simulink model "test_simulink"  (R2017a)
settings: Solver=VariableStepAuto  StartTime=0.0  StopTime=10.0  RelTol=1e-3
values from neighbouring files (symbols this model uses):
  ddq = u(15:21)    [accelerations_simulink.m]    (also in comparison_simulink.m = ADAMS_yout(:,37:43); gravity_force_simulink.m; gravity_moment_simulink.m; inertia_force_simulink.m)
settings Model: Creator=ashwi  LastModifiedBy=ashwi

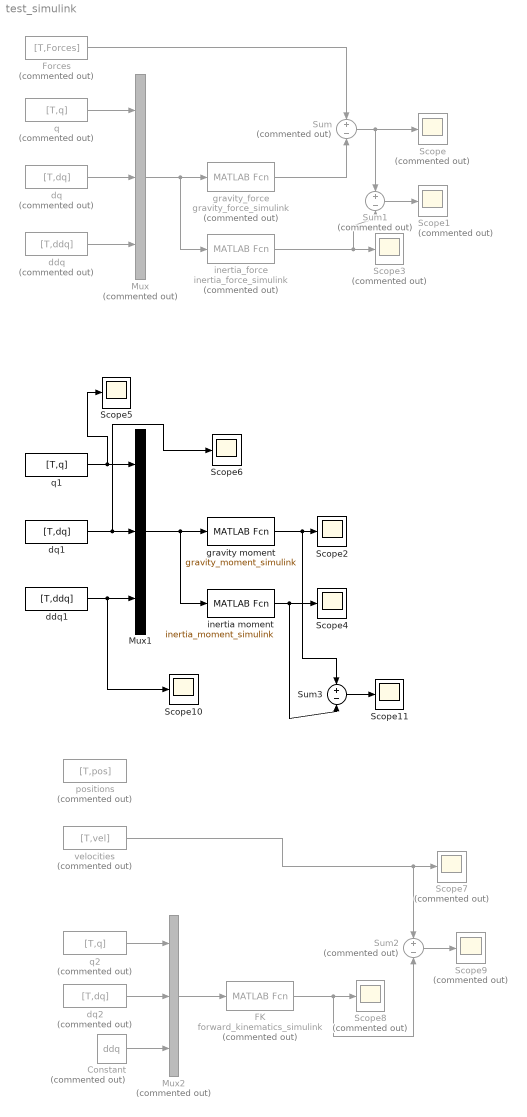
== system test_simulink ==
  Constant : Constant  Commented=on  Value=ddq
  FK : MATLABFcn  Commented=on  MATLABFcn=forward_kinematics_simulink
  Forces : FromWorkspace  Commented=on  VariableName=[T,Forces]  SampleTime=0
  Mux : Mux  Commented=on  Inputs=3
  Mux1 : Mux  Inputs=3
  Mux2 : Mux  Commented=on  Inputs=3
  Scope{,1,3,7..9} (6 alike) : Scope  Commented=on
  Scope{2,4..6,10..11} (6 alike) : Scope
  Sum : Sum  Commented=on  Inputs=+-
  Sum1 : Sum  Commented=on  Inputs=+-
  Sum2 : Sum  Commented=on  Inputs=+-
  Sum3 : Sum  Inputs=+-
  ddq : FromWorkspace  Commented=on  VariableName=[T,ddq]  SampleTime=0
  ddq1 : FromWorkspace  VariableName=[T,ddq]  SampleTime=0
  dq : FromWorkspace  Commented=on  VariableName=[T,dq]  SampleTime=0
  dq1 : FromWorkspace  VariableName=[T,dq]  SampleTime=0
  dq2 : FromWorkspace  Commented=on  VariableName=[T,dq]  SampleTime=0
  gravity moment : MATLABFcn  MATLABFcn=gravity_moment_simulink
  gravity_force : MATLABFcn  Commented=on  MATLABFcn=gravity_force_simulink
  inertia moment : MATLABFcn  MATLABFcn=inertia_moment_simulink
  inertia_force : MATLABFcn  Commented=on  MATLABFcn=inertia_force_simulink
  positions : FromWorkspace  Commented=on  VariableName=[T,pos]  SampleTime=0
  q : FromWorkspace  Commented=on  VariableName=[T,q]  SampleTime=0
  q1 : FromWorkspace  VariableName=[T,q]  SampleTime=0
  q2 : FromWorkspace  Commented=on  VariableName=[T,q]  SampleTime=0
  velocities : FromWorkspace  Commented=on  VariableName=[T,vel]  SampleTime=0
  wires:
  Mux/1 -> inertia_force/1, gravity_force/1
  dq/1 -> Mux/2
  q/1 -> Mux/1
  ddq/1 -> Mux/3
  gravity_force/1 -> Sum/2
  Forces/1 -> Sum/1
  Sum/1 -> Sum1/1, Scope/1
  inertia_force/1 -> Sum1/2, Scope3/1
  Sum1/1 -> Scope1/1
  q1/1 -> Scope5/1, Mux1/1
  dq1/1 -> Scope6/1, Mux1/2
  ddq1/1 -> Scope10/1, Mux1/3
  Mux1/1 -> inertia moment/1, gravity moment/1
  gravity moment/1 -> Sum3/1, Scope2/1
  inertia moment/1 -> Sum3/2, Scope4/1
  q2/1 -> Mux2/1
  dq2/1 -> Mux2/2
  Constant/1 -> Mux2/3
  Mux2/1 -> FK/1
  FK/1 -> Sum2/2, Scope8/1
  Sum2/1 -> Scope9/1
  velocities/1 -> Sum2/1, Scope7/1
  Sum3/1 -> Scope11/1
